simulink model "CoherenceCalculation"  (R2016b)
settings: Solver=FixedStepDiscrete  StartTime=0.0  StopTime=inf  FixedStep=sCoreParams.core.stepPeriod  RelTol=1e-3  EnableMultiTasking=on
undefined symbols (not defined in the file): sCoreParams
settings Model: Creator=anish  LastModifiedBy=rzelmann
settings SolverCC: EnableConcurrentExecution=on  ConcurrentTasks=on
settings DataIOCC: SaveFormat=StructureWithTime  SignalLoggingSaveFormat=ModelDataLogs  SaveOutput=off  SignalLogging=off  DSMLogging=off  SaveTime=off
settings OptimizationCC: BlockReduction=off  ConditionallyExecuteInputs=off  DefaultParameterBehavior=Inlined  OptimizeBlockIOStorage=off  BufferReuse=off  GlobalBufferReuse=off  ExpressionFolding=off  LocalBlockOutputs=off  LifeSpan=inf
settings DebuggingCC: SignalRangeChecking=error  SaveWithParameterizedLinksMsg=none  AllowSymbolicDim=off  ModelReferenceSymbolNameMessage=none  StateNameClashWarn=warning  SFUnexpectedBacktrackingDiag=warning  SFNoUnconditionalDefaultTransitionDiag=warning  SFExecutionAtInitializationDiag=none
settings HardwareCC: ProdBitPerPointer=32  ProdBitPerSizeT=32  ProdBitPerPtrDiffT=32  ProdLargestAtomicFloat=None  ProdWordSize=32  ProdLongLongMode=on  ProdHWDeviceType=Generic->32-bit x86 compatible  TargetBitPerPointer=64  TargetLargestAtomicFloat=Float  TargetLongLongMode=on  TargetIntDivRoundTo=Zero  TargetEndianess=LittleEndian  TargetWordSize=64  TargetHWDeviceType=Intel->x86-64 (Windows64)
settings ModelReferenceCC: UpdateModelReferenceTargets=Force  ModelReferenceNumInstancesAllowed=Single  ModelReferencePassRootInputsByReference=off
settings RTWCC: SystemTargetFile=slrt.tlc  TemplateMakefile=slrt_default_tmf  Description=Simulink Real-Time  BuildConfiguration=Faster Runs  RTWCompilerOptimization=on
settings TargetCC: CodeReplacementLibrary=XPC_BLAS  ParMdlRefBuildCompliant=on  ConcurrentExecutionCompliant=on  GeneratePreprocessorConditionals=Use local settings  MatFileLogging=on  MATLABClassNameForMDSCustomization=xpcAperiodicCustomization
settings ConfigComp: CovMetricSettings=dw  CovHtmlReporting=on  CovSaveCumulativeToWorkspaceVar=on  CovSaveSingleToWorkspaceVar=on  CovExternalEMLEnable=off  CovSFcnEnable=off

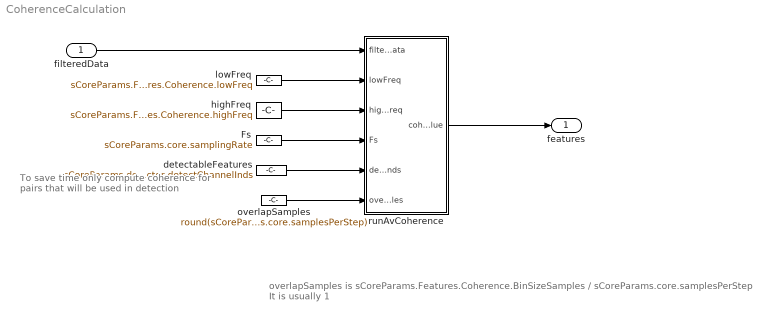
== system CoherenceCalculation ==
  note: overlapSamples is  sCoreParams.Features.Coherence.BinSizeSamples / sCoreParams.core.samplesPerStep
      | It is usually 1
  note: To save time only compute coherence
      | for pairs that will be used in detection
  filteredData : Inport  PortDimensions=[sCoreParams.Features.Coherence.WindowDurationSamples sCoreParams.decoders.txDetector.nFilteredChannels]
  Fs : Constant  Value=sCoreParams.core.samplingRate
  detectableFeatures : Constant  Value=sCoreParams.decoders.txDetector.detectChannelInds
  highFreq : Constant  Value=sCoreParams.Features.Coherence.highFreq
  lowFreq : Constant  Value=sCoreParams.Features.Coherence.lowFreq
  overlapSamples : Constant  Value=round(sCoreParams.Features.Coherence.BinSizeSamples/sCoreParams.core.samplesPerStep)
  runAvCoherence : MATLAB Function  TreatAsAtomicUnit=on
  features : Outport
  wires:
  runAvCoherence/1(coherenceValue) -> features/1
  lowFreq/1 -> runAvCoherence/2(lowFreq)
  highFreq/1 -> runAvCoherence/3(highFreq)
  Fs/1 -> runAvCoherence/4(Fs)
  filteredData/1 -> runAvCoherence/1(filteredData)
  detectableFeatures/1 -> runAvCoherence/5(detectPairInds)
  overlapSamples/1 -> runAvCoherence/6(overlapSamples)

== matlab function CoherenceCalculation/runAvCoherence ==
  data: filteredData input; coherenceValue output; lowFreq input; highFreq input; Fs input; detectPairInds input; overlapSamples input
function coherenceValue   = runCoherence(filteredData,  lowFreq, highFreq, Fs, detectPairInds, overlapSamples)
%#codegen
% Run mscohere in filteredData
% Returns magnitude-square coherence between pairs of channels for the whole time window
% coder.extrinsic('mscohere');
% freqBins = linspace(lowFreq, highFreq, 64);
% [coherenceValue1, fValues] = mscohere(filteredData, filteredData, [], [], freqBins, Fs);
% avCoherence1 = mean(coherenceValue1(:));    % average across all intereactions

%[~, avCoherence, coherenceValue, pairChannels] = runCoherence_EML(filteredData, lowFreq, highFreq, Fs, detectPairInds, overlapSamples);
%    [coherenceValue] = runCoherence_NoDownsampling_EML(filteredData, lowFreq, highFreq, Fs, detectPairInds, overlapSamples);
    [coherenceValue] = runCoherence_MatrixForm_NoDownsampling_EML(filteredData, lowFreq, highFreq, Fs, detectPairInds, overlapSamples); % to use multiple cores compute Pxy as a mtraix for ALL pairs

%[sumCoherencePerChannel, avCoherence, coherenceValue] = runCoherenceMultitaper_EML(filteredData, lowFreq, highFreq, nPoints, Fs);
